simulink model "trajectory_test"  (Simulink 6.4)
settings: Solver=ode4  StartTime=0.0  StopTime=20  FixedStep=0.01  RelTol=1e-3
values from neighbouring files (symbols this model uses):
  trajectory_time = 2    [param_list.m]
undefined symbols (not defined in the file or in its folder): DiscIntNeverNeededParam
libraries: simulink x3
settings Model: LastModifiedBy=Developer

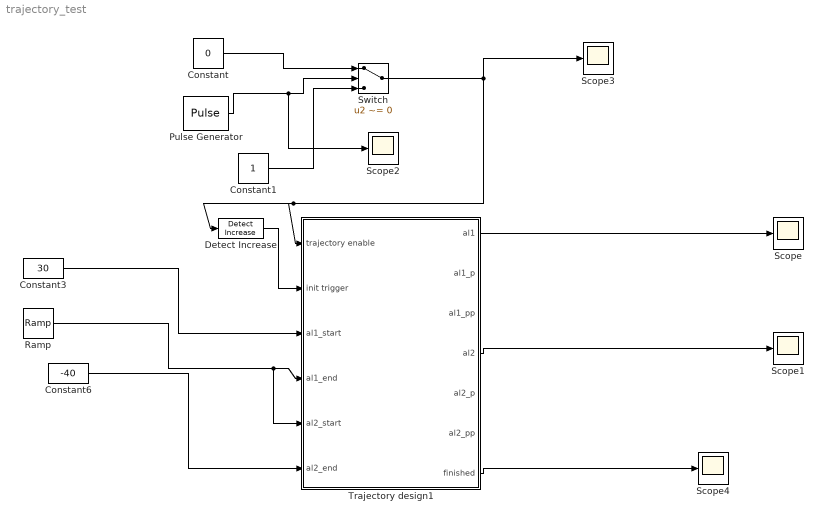
== system trajectory_test ==
  Constant : Constant  Value=0  OutDataType=sfix(16)  ConRadixGroup=Use specified scaling  OutScaling=2^0  SampleTime=inf  FramePeriod=inf
  Constant1 : Constant  Value=1  OutDataType=sfix(16)  ConRadixGroup=Use specified scaling  OutScaling=2^0  SampleTime=inf  FramePeriod=inf
  Constant3 : Constant  Value=30  OutDataType=sfix(16)  ConRadixGroup=Use specified scaling  OutScaling=2^0  SampleTime=inf  FramePeriod=inf
  Constant6 : Constant  Value=-40  OutDataType=sfix(16)  ConRadixGroup=Use specified scaling  OutScaling=2^0  SampleTime=inf  FramePeriod=inf
  Detect Increase : simulink/Logic and Bit Operations/Detect Increase  SystemSampleTime=-1  vinit=0.0
  Pulse Generator : DiscretePulseGenerator  PulseType=Time based  Period=6  PulseWidth=50
  Ramp : simulink/Sources/Ramp  SystemSampleTime=-1  slope=1  start=0  X0=0
  Scope{,1..4} (5 alike) : Scope
      Scope settings: YMin=38  YMax=42
      Scope2 settings: YMin=38  YMax=42  SaveName=ScopeData2
      Scope3 settings: YMin=38  YMax=42  SaveName=ScopeData3
      Scope4 settings: SaveName=ScopeData4
  Switch : Switch  Criteria=u2 ~= 0
  Trajectory design1 : Subsystem
  wires:
  Switch/1 -> Scope3/1, Detect Increase/1, Trajectory design1/1(trajectory enable)
  Constant/1 -> Switch/1
  Pulse Generator/1 -> Switch/2, Scope2/1
  Constant1/1 -> Switch/3
  Detect Increase/1 -> Trajectory design1/2(init trigger)
  Constant3/1 -> Trajectory design1/3(al1_start)
  Ramp/1 -> Trajectory design1/5(al2_start), Trajectory design1/4(al1_end)
  Constant6/1 -> Trajectory design1/6(al2_end)
  Trajectory design1/1(al1) -> Scope/1
  Trajectory design1/4(al2) -> Scope1/1
  Trajectory design1/7(finished) -> Scope4/1

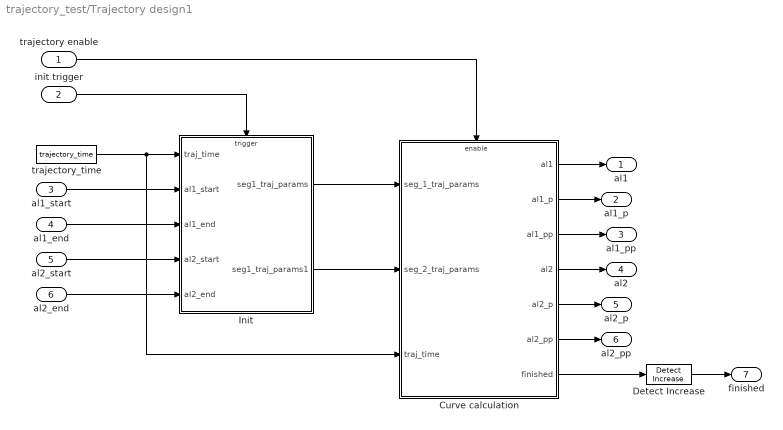
== system trajectory_test/Trajectory design1 ==
  trajectory enable : Inport
  init trigger : Inport  Port=2
  al1_start : Inport  Port=3
  al1_end : Inport  Port=4
  al2_start : Inport  Port=5
  al2_end : Inport  Port=6
  Curve calculation : Subsystem
  Detect Increase : simulink/Logic and Bit Operations/Detect Increase  SystemSampleTime=-1  vinit=0.0
  Init : Subsystem
  trajectory_time : Constant  Value=trajectory_time  OutDataType=sfix(16)  ConRadixGroup=Use specified scaling  OutScaling=2^0  SampleTime=inf  FramePeriod=inf
  al1 : Outport
  al1_p : Outport  Port=2
  al1_pp : Outport  Port=3
  al2 : Outport  Port=4
  al2_p : Outport  Port=5
  al2_pp : Outport  Port=6
  finished : Outport  Port=7
  wires:
  trajectory_time/1 -> Curve calculation/3(traj_time), Init/1(traj_time)
  al1_end/1 -> Init/3(al1_end)
  Init/2(seg1_traj_params1) -> Curve calculation/2(seg_2_traj_params)
  Init/1(seg1_traj_params) -> Curve calculation/1(seg_1_traj_params)
  trajectory enable/1 -> Curve calculation/Enable
  Curve calculation/1(al1) -> al1/1
  Curve calculation/2(al1_p) -> al1_p/1
  al1_start/1 -> Init/2(al1_start)
  Curve calculation/3(al1_pp) -> al1_pp/1
  Curve calculation/4(al2) -> al2/1
  Curve calculation/5(al2_p) -> al2_p/1
  Curve calculation/6(al2_pp) -> al2_pp/1
  al2_start/1 -> Init/4(al2_start)
  al2_end/1 -> Init/5(al2_end)
  init trigger/1 -> Init/Trigger
  Curve calculation/7(finished) -> Detect Increase/1
  Detect Increase/1 -> finished/1

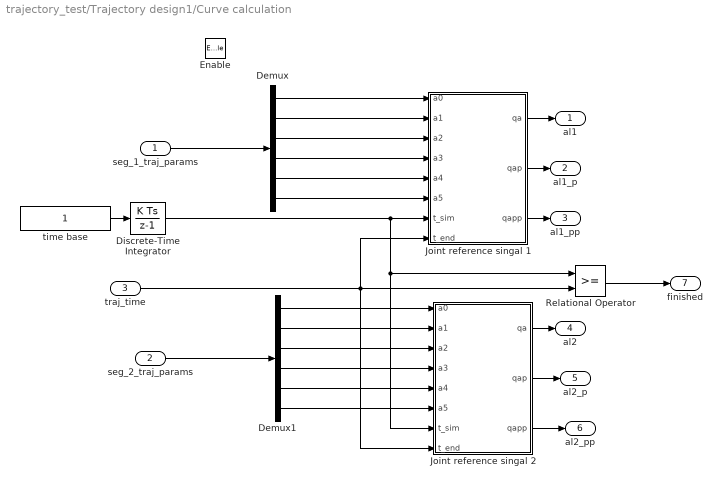
== system trajectory_test/Trajectory design1/Curve calculation ==
  seg_1_traj_params : Inport
  seg_2_traj_params : Inport  Port=2
  traj_time : Inport  Port=3
  Enable : EnablePort  StatesWhenEnabling=reset
  Demux : Demux  Outputs=6
  Demux1 : Demux  Outputs=6
  Discrete-Time Integrator : DiscreteIntegrator  SampleTime=-1  ICPrevOutput=DiscIntNeverNeededParam  ICPrevScaledInput=DiscIntNeverNeededParam
  Joint reference singal 1 : Stateflow chart  TreatAsAtomicUnit=on
  Joint reference singal 2 : Stateflow chart  TreatAsAtomicUnit=on
  Relational Operator : RelationalOperator  LogicOutDataTypeMode=Boolean
  time base : Constant  Value=1  OutDataType=sfix(16)  ConRadixGroup=Use specified scaling  OutScaling=2^0  SampleTime=inf  FramePeriod=inf
  al1 : Outport
  al1_p : Outport  Port=2
  al1_pp : Outport  Port=3
  al2 : Outport  Port=4
  al2_p : Outport  Port=5
  al2_pp : Outport  Port=6
  finished : Outport  Port=7
  wires:
  Joint reference singal 1/1(qa) -> al1/1
  Joint reference singal 1/2(qap) -> al1_p/1
  Joint reference singal 1/3(qapp) -> al1_pp/1
  Joint reference singal 2/1(qa) -> al2/1
  Discrete-Time Integrator/1 -> Joint reference singal 1/7(t_sim), Joint reference singal 2/7(t_sim), Relational Operator/1
  time base/1 -> Discrete-Time Integrator/1
  Demux/1 -> Joint reference singal 1/1(a0)
  Demux/2 -> Joint reference singal 1/2(a1)
  Demux/3 -> Joint reference singal 1/3(a2)
  Demux/4 -> Joint reference singal 1/4(a3)
  Demux/5 -> Joint reference singal 1/5(a4)
  Demux/6 -> Joint reference singal 1/6(a5)
  Demux1/1 -> Joint reference singal 2/1(a0)
  Demux1/2 -> Joint reference singal 2/2(a1)
  Demux1/3 -> Joint reference singal 2/3(a2)
  Demux1/4 -> Joint reference singal 2/4(a3)
  Demux1/5 -> Joint reference singal 2/5(a4)
  Demux1/6 -> Joint reference singal 2/6(a5)
  seg_1_traj_params/1 -> Demux/1
  seg_2_traj_params/1 -> Demux1/1
  traj_time/1 -> Joint reference singal 1/8(t_end), Joint reference singal 2/8(t_end), Relational Operator/2
  Relational Operator/1 -> finished/1
  Joint reference singal 2/2(qap) -> al2_p/1
  Joint reference singal 2/3(qapp) -> al2_pp/1

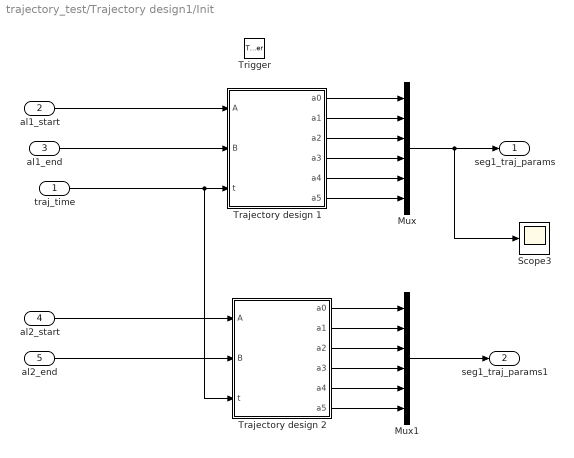
== system trajectory_test/Trajectory design1/Init ==
  traj_time : Inport
  al1_start : Inport  Port=2  LatchByDelayingOutsideSignal=on
  al1_end : Inport  Port=3
  al2_start : Inport  Port=4  LatchByDelayingOutsideSignal=on
  al2_end : Inport  Port=5
  Trigger : TriggerPort
  Mux : Mux  Inputs=6
  Mux1 : Mux  Inputs=6
  Scope3 : Scope
      settings: YMin=38  YMax=42  SaveName=ScopeData5
  Trajectory design 1 : Stateflow chart  TreatAsAtomicUnit=on
  Trajectory design 2 : Stateflow chart  TreatAsAtomicUnit=on
  seg1_traj_params : Outport
  seg1_traj_params1 : Outport  Port=2
  wires:
  al1_start/1 -> Trajectory design 1/1(A)
  al1_end/1 -> Trajectory design 1/2(B)
  al2_start/1 -> Trajectory design 2/1(A)
  al2_end/1 -> Trajectory design 2/2(B)
  traj_time/1 -> Trajectory design 1/3(t), Trajectory design 2/3(t)
  Trajectory design 1/1(a0) -> Mux/1
  Trajectory design 1/2(a1) -> Mux/2
  Trajectory design 1/3(a2) -> Mux/3
  Trajectory design 1/4(a3) -> Mux/4
  Trajectory design 1/5(a4) -> Mux/5
  Trajectory design 1/6(a5) -> Mux/6
  Trajectory design 2/1(a0) -> Mux1/1
  Trajectory design 2/2(a1) -> Mux1/2
  Trajectory design 2/3(a2) -> Mux1/3
  Trajectory design 2/4(a3) -> Mux1/4
  Trajectory design 2/5(a4) -> Mux1/5
  Trajectory design 2/6(a5) -> Mux1/6
  Mux/1 -> seg1_traj_params/1, Scope3/1
  Mux1/1 -> seg1_traj_params1/1

== matlab function Trajectory design1/Curve calculation/Joint reference singal 1 ==
  data: a0 input double; a1 input double; a2 input double; a3 input double; a4 input double; a5 input double; t_sim input double; qa output double; qap output double; qapp output double; t_end input double
function [qa,qap,qapp] = fcn(a0,a1,a2,a3,a4,a5,t_sim,t_end)
% This block supports an embeddable subset of the MATLAB language.
% See the help menu for details. 
if (t_sim>=t_end) 
    t_sim = t_end;
end   
T = [t_sim^5/20 t_sim^4/12 t_sim^3/6 t_sim^2/2 t_sim 1;...
    t_sim^4/4 t_sim^3/3 t_sim^2/2 t_sim 1 0;...
    t_sim^3 t_sim^2 t_sim 1 0 0];
Q = T*[a0;a1;a2;a3;a4;a5];

qa = Q(1);
qap = Q(2);
qapp = Q(3);

== matlab function Trajectory design1/Curve calculation/Joint reference singal 2 ==
  data: a0 input double; a1 input double; a2 input double; a3 input double; a4 input double; a5 input double; t_sim input double; qa output double; qap output double; qapp output double; t_end input double
function [qa,qap,qapp] = fcn(a0,a1,a2,a3,a4,a5,t_sim,t_end)
% This block supports an embeddable subset of the MATLAB language.
% See the help menu for details. 
if (t_sim>=t_end) 
    t_sim = t_end;
end   
T = [t_sim^5/20 t_sim^4/12 t_sim^3/6 t_sim^2/2 t_sim 1;...
    t_sim^4/4 t_sim^3/3 t_sim^2/2 t_sim 1 0;...
    t_sim^3 t_sim^2 t_sim 1 0 0];
Q = T*[a0;a1;a2;a3;a4;a5];

qa = Q(1);
qap = Q(2);
qapp = Q(3);

== matlab function Trajectory design1/Init/Trajectory design 1 ==
  data: A input double; B input double; t input double; a0 output double; a1 output double; a2 output double; a3 output double; a4 output double; a5 output double
function [a0,a1,a2,a3,a4,a5] = fcn(A,B,t)
% This block supports an embeddable subset of the MATLAB language.
% See the help menu for details. 
T = [t^5/20 t^4/12 t^3/6 t^2/2 t 1;t^4/4 t^3/3 t^2/2 t 1 0;t^3 t^2 t 1 0 0;0 0 0 0 0 1;0 0 0 0 1 0;0 0 0 1 0 0];
Ao = inv(T)*[B;0;0;A;0;0];
a0=Ao(1);
a1=Ao(2);
a2=Ao(3);
a3=Ao(4);
a4=Ao(5);
a5=Ao(6);

== matlab function Trajectory design1/Init/Trajectory design 2 ==
  data: A input double; B input double; t input double; a0 output double; a1 output double; a2 output double; a3 output double; a4 output double; a5 output double
function [a0,a1,a2,a3,a4,a5] = fcn(A,B,t)
% This block supports an embeddable subset of the MATLAB language.
% See the help menu for details. 
T = [t^5/20 t^4/12 t^3/6 t^2/2 t 1;t^4/4 t^3/3 t^2/2 t 1 0;t^3 t^2 t 1 0 0;0 0 0 0 0 1;0 0 0 0 1 0;0 0 0 1 0 0];
Ao = inv(T)*[B;0;0;A;0;0];
a0=Ao(1);
a1=Ao(2);
a2=Ao(3);
a3=Ao(4);
a4=Ao(5);
a5=Ao(6);
